simulink model "Physical_architecture"  (R2023b)
settings: Solver=VariableStepAuto  StartTime=0.0  StopTime=10.0  RelTol=1e-3
settings Model: Creator=Cristian  LastModifiedBy=Cristian

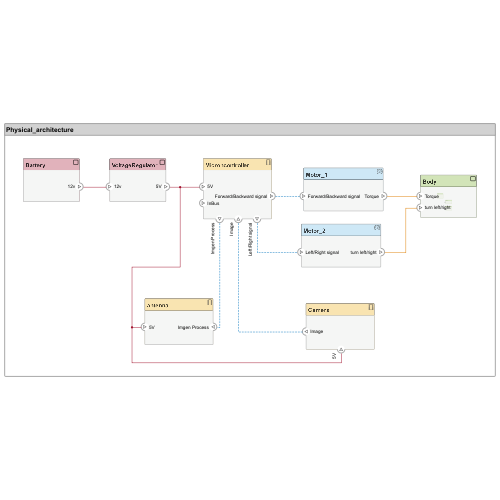
[thumbnail: Simulink's stored preview of the top-level diagram]
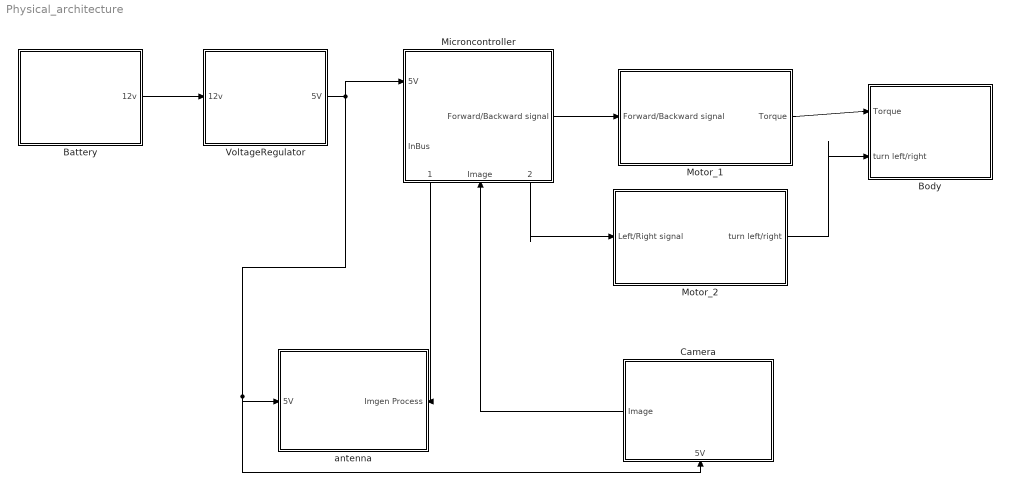
== system Physical_architecture ==
  Battery : Subsystem
      settings: PortSchema="{\"entries\":[{\"content\":{\"headerSize\":26,\"margin\":15,\"minimumSpacing\":25,\"sides\":[{\"content\":{},\"type\":\"ConnectorPlacement.EquallySpacedRectSide\",\"uuid\":\"a4c63610-ce53-4263-bc32-11f7e141828d\"},{\"content\":{\"connectorIds\":[\"Out1\"],\"side\":\"RIGHT\"},\"type\":\"ConnectorPlacement.EquallySpacedRectSide\",\"uuid\":\"7388023e-6661-4314-a5ba-fe6a68600945\"},{\"content\":{\"side\":\"TOP\"},\"type\":\"ConnectorPlacement.EquallySpacedRectSide\",\"uuid\":\"a8a6465a-b279-4272-9cd6-de33cf491c4f\"}]},\"type\":\"ConnectorPlacement.EquallySpacedConnector\",\"uuid\":\"83902977-a181-41b3-bc45-d69d98624d59\"}],\"packageUris\":[\"http://schema.mathworks.com/mf0/Connector/R2020b\"],\"version\":\"1.0\"}"
  Body : Subsystem
      settings: PortSchema="{\"entries\":[{\"content\":{\"headerSize\":26,\"margin\":15,\"minimumSpacing\":25,\"sides\":[{\"content\":{\"connectorIds\":[\"In2\",\"In1\"]},\"type\":\"ConnectorPlacement.EquallySpacedRectSide\",\"uuid\":\"a4c63610-ce53-4263-bc32-11f7e141828d\"},{\"content\":{\"side\":\"RIGHT\"},\"type\":\"ConnectorPlacement.EquallySpacedRectSide\",\"uuid\":\"7388023e-6661-4314-a5ba-fe6a68600945\"},{\"content\":{\"side\":\"TOP\"},\"type\":\"ConnectorPlacement.EquallySpacedRectSide\",\"uuid\":\"a8a6465a-b279-4272-9cd6-de33cf491c4f\"},{\"content\":{\"side\":\"BOTTOM\"},\"type\":\"ConnectorPlacement.EquallySpacedRectSide\",\"uuid\":\"22874e39-900b-4eaf-ad8f-1ca0f898979d\"}]},\"type\":\"ConnectorPlacement.EquallySpacedConnector\",\"uuid\":\"83902977-a181-41b3-bc45-d69d98624d59\"}],\"packageUris\":[\"http://schema.mathworks.com/mf0/Connector/R2020b\"],\"version\":\"1.0\"}"
  Camera : Subsystem
      settings: PortSchema="{\"entries\":[{\"content\":{\"headerSize\":26,\"margin\":15,\"minimumSpacing\":25,\"sides\":[{\"content\":{\"connectorIds\":[\"Out1\"]},\"type\":\"ConnectorPlacement.EquallySpacedRectSide\",\"uuid\":\"a4c63610-ce53-4263-bc32-11f7e141828d\"},{\"content\":{\"side\":\"RIGHT\"},\"type\":\"ConnectorPlacement.EquallySpacedRectSide\",\"uuid\":\"7388023e-6661-4314-a5ba-fe6a68600945\"},{\"content\":{\"side\":\"TOP\"},\"type\":\"ConnectorPlacement.EquallySpacedRectSide\",\"uuid\":\"a8a6465a-b279-4272-9cd6-de33cf491c4f\"},{\"content\":{\"connectorIds\":[\"In1\"],\"side\":\"BOTTOM\"},\"type\":\"ConnectorPlacement.EquallySpacedRectSide\",\"uuid\":\"23249c11-1fad-4353-8010-062f6ccc5b3b\"}]},\"type\":\"ConnectorPlacement.EquallySpacedConnector\",\"uuid\":\"83902977-a181-41b3-bc45-d69d98624d59\"}],\"packageUris\":[\"http://schema.mathworks.com/mf0/Connector/R2020b\"],\"version\":\"1.0\"}"
  Microncontroller : Subsystem
      settings: PortSchema="{\"entries\":[{\"content\":{\"headerSize\":26,\"margin\":15,\"minimumSpacing\":25,\"sides\":[{\"content\":{\"connectorIds\":[\"In2\",\"In3\"]},\"type\":\"ConnectorPlacement.EquallySpacedRectSide\",\"uuid\":\"a4c63610-ce53-4263-bc32-11f7e141828d\"},{\"content\":{\"connectorIds\":[\"Out3\"],\"side\":\"RIGHT\"},\"type\":\"ConnectorPlacement.EquallySpacedRectSide\",\"uuid\":\"7388023e-6661-4314-a5ba-fe6a68600945\"},{\"content\":{\"side\":\"TOP\"},\"type\":\"ConnectorPlacement.EquallySpacedRectSide\",\"uuid\":\"a8a6465a-b279-4272-9cd6-de33cf491c4f\"},{\"content\":{\"connectorIds\":[\"Out1\",\"In1\",\"Out2\"],\"side\":\"BOTTOM\"},\"type\":\"ConnectorPlacement.EquallySpacedRectSide\",\"uuid\":\"9aefb96e-8b5c-4ea9-bd4f-4224df175b07\"}]},\"type\":\"ConnectorPlacement.EquallySpacedConnector\",\"uuid\":\"83902977-a181-41b3-bc45-d69d98624d59\"}],\"packageUris\":[\"http://schema.mathworks.com/mf0/Connector/R2020b\"],\"version\":\"1.0\"}"
  Motor_1 : Subsystem
      settings: PortSchema="{\"entries\":[{\"content\":{\"headerSize\":26,\"margin\":15,\"minimumSpacing\":25,\"sides\":[{\"content\":{\"connectorIds\":[\"In1\"]},\"type\":\"ConnectorPlacement.EquallySpacedRectSide\",\"uuid\":\"a4c63610-ce53-4263-bc32-11f7e141828d\"},{\"content\":{\"connectorIds\":[\"Out1\"],\"side\":\"RIGHT\"},\"type\":\"ConnectorPlacement.EquallySpacedRectSide\",\"uuid\":\"7388023e-6661-4314-a5ba-fe6a68600945\"},{\"content\":{\"side\":\"TOP\"},\"type\":\"ConnectorPlacement.EquallySpacedRectSide\",\"uuid\":\"a8a6465a-b279-4272-9cd6-de33cf491c4f\"}]},\"type\":\"ConnectorPlacement.EquallySpacedConnector\",\"uuid\":\"83902977-a181-41b3-bc45-d69d98624d59\"}],\"packageUris\":[\"http://schema.mathworks.com/mf0/Connector/R2020b\"],\"version\":\"1.0\"}"
  Motor_2 : Subsystem
      settings: PortSchema="{\"entries\":[{\"content\":{\"headerSize\":26,\"margin\":15,\"minimumSpacing\":25,\"sides\":[{\"content\":{\"connectorIds\":[\"In1\"]},\"type\":\"ConnectorPlacement.EquallySpacedRectSide\",\"uuid\":\"a4c63610-ce53-4263-bc32-11f7e141828d\"},{\"content\":{\"connectorIds\":[\"Out1\"],\"side\":\"RIGHT\"},\"type\":\"ConnectorPlacement.EquallySpacedRectSide\",\"uuid\":\"7388023e-6661-4314-a5ba-fe6a68600945\"},{\"content\":{\"side\":\"TOP\"},\"type\":\"ConnectorPlacement.EquallySpacedRectSide\",\"uuid\":\"a8a6465a-b279-4272-9cd6-de33cf491c4f\"}]},\"type\":\"ConnectorPlacement.EquallySpacedConnector\",\"uuid\":\"83902977-a181-41b3-bc45-d69d98624d59\"}],\"packageUris\":[\"http://schema.mathworks.com/mf0/Connector/R2020b\"],\"version\":\"1.0\"}"
  VoltageRegulator : Subsystem
      settings: PortSchema="{\"entries\":[{\"content\":{\"headerSize\":26,\"margin\":15,\"minimumSpacing\":25,\"sides\":[{\"content\":{\"connectorIds\":[\"In1\"]},\"type\":\"ConnectorPlacement.EquallySpacedRectSide\",\"uuid\":\"a4c63610-ce53-4263-bc32-11f7e141828d\"},{\"content\":{\"connectorIds\":[\"Out1\"],\"side\":\"RIGHT\"},\"type\":\"ConnectorPlacement.EquallySpacedRectSide\",\"uuid\":\"7388023e-6661-4314-a5ba-fe6a68600945\"},{\"content\":{\"side\":\"TOP\"},\"type\":\"ConnectorPlacement.EquallySpacedRectSide\",\"uuid\":\"a8a6465a-b279-4272-9cd6-de33cf491c4f\"}]},\"type\":\"ConnectorPlacement.EquallySpacedConnector\",\"uuid\":\"83902977-a181-41b3-bc45-d69d98624d59\"}],\"packageUris\":[\"http://schema.mathworks.com/mf0/Connector/R2020b\"],\"version\":\"1.0\"}"
  antenna : Subsystem
      settings: PortSchema="{\"entries\":[{\"content\":{\"headerSize\":26,\"margin\":15,\"minimumSpacing\":25,\"sides\":[{\"content\":{\"connectorIds\":[\"In2\"]},\"type\":\"ConnectorPlacement.EquallySpacedRectSide\",\"uuid\":\"a4c63610-ce53-4263-bc32-11f7e141828d\"},{\"content\":{\"connectorIds\":[\"In1\"],\"side\":\"RIGHT\"},\"type\":\"ConnectorPlacement.EquallySpacedRectSide\",\"uuid\":\"7388023e-6661-4314-a5ba-fe6a68600945\"},{\"content\":{\"side\":\"TOP\"},\"type\":\"ConnectorPlacement.EquallySpacedRectSide\",\"uuid\":\"a8a6465a-b279-4272-9cd6-de33cf491c4f\"}]},\"type\":\"ConnectorPlacement.EquallySpacedConnector\",\"uuid\":\"83902977-a181-41b3-bc45-d69d98624d59\"}],\"packageUris\":[\"http://schema.mathworks.com/mf0/Connector/R2020b\"],\"version\":\"1.0\"}"
  wires:
  Battery/1(12v) -> VoltageRegulator/1(12v)
  VoltageRegulator/1(5V) -> antenna/2(5V), Camera/1(5V), Microncontroller/2(5V)
  Microncontroller/3(Forward/Backward signal) -> Motor_1/1(Forward/Backward signal)
  Microncontroller/2(Left/Right signal) -> Motor_2/1(Left/Right signal)
  Motor_1/1(Torque) -> Body/2(Torque)
  Motor_2/1(turn left/right) -> Body/1(turn left/right)
  Camera/1(Image) -> Microncontroller/1(Image)
  Microncontroller/1(Imgen Process) -> antenna/1(Imgen Process)

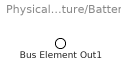
== system Physical_architecture/Battery ==
  Bus Element Out1 : Outport  PortName=12v

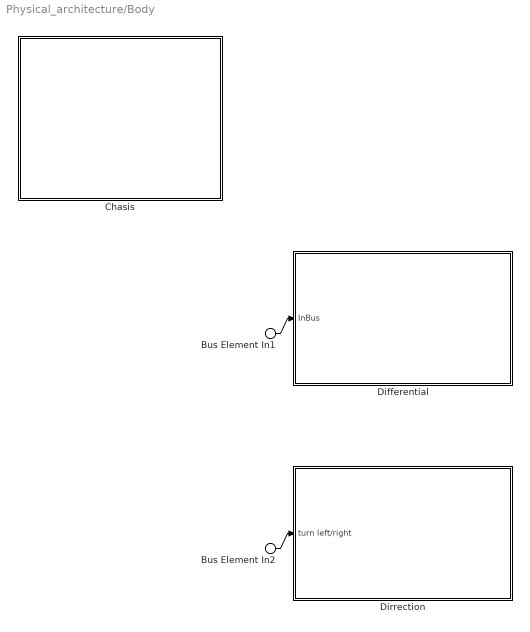
== system Physical_architecture/Body ==
  Bus Element In2 : Inport  PortName=turn left/right
  Bus Element In1 : Inport  Port=2  PortName=Torque
  Chasis : Subsystem
      settings: PortSchema="{\"entries\":[{\"content\":{\"headerSize\":26,\"margin\":15,\"minimumSpacing\":25,\"sides\":[{\"content\":{},\"type\":\"ConnectorPlacement.EquallySpacedRectSide\",\"uuid\":\"a4c63610-ce53-4263-bc32-11f7e141828d\"},{\"content\":{\"side\":\"RIGHT\"},\"type\":\"ConnectorPlacement.EquallySpacedRectSide\",\"uuid\":\"7388023e-6661-4314-a5ba-fe6a68600945\"},{\"content\":{\"side\":\"TOP\"},\"type\":\"ConnectorPlacement.EquallySpacedRectSide\",\"uuid\":\"a8a6465a-b279-4272-9cd6-de33cf491c4f\"}]},\"type\":\"ConnectorPlacement.EquallySpacedConnector\",\"uuid\":\"83902977-a181-41b3-bc45-d69d98624d59\"}],\"packageUris\":[\"http://schema.mathworks.com/mf0/Connector/R2020b\"],\"version\":\"1.0\"}"
  Differential : Subsystem
      settings: PortSchema="{\"entries\":[{\"content\":{\"headerSize\":26,\"margin\":15,\"minimumSpacing\":25,\"sides\":[{\"content\":{\"connectorIds\":[\"In1\"]},\"type\":\"ConnectorPlacement.EquallySpacedRectSide\",\"uuid\":\"a4c63610-ce53-4263-bc32-11f7e141828d\"},{\"content\":{\"side\":\"RIGHT\"},\"type\":\"ConnectorPlacement.EquallySpacedRectSide\",\"uuid\":\"7388023e-6661-4314-a5ba-fe6a68600945\"},{\"content\":{\"side\":\"TOP\"},\"type\":\"ConnectorPlacement.EquallySpacedRectSide\",\"uuid\":\"a8a6465a-b279-4272-9cd6-de33cf491c4f\"}]},\"type\":\"ConnectorPlacement.EquallySpacedConnector\",\"uuid\":\"83902977-a181-41b3-bc45-d69d98624d59\"}],\"packageUris\":[\"http://schema.mathworks.com/mf0/Connector/R2020b\"],\"version\":\"1.0\"}"
  Dirrection : Subsystem
      settings: PortSchema="{\"entries\":[{\"content\":{\"headerSize\":26,\"margin\":15,\"minimumSpacing\":25,\"sides\":[{\"content\":{\"connectorIds\":[\"In1\"]},\"type\":\"ConnectorPlacement.EquallySpacedRectSide\",\"uuid\":\"a4c63610-ce53-4263-bc32-11f7e141828d\"},{\"content\":{\"side\":\"RIGHT\"},\"type\":\"ConnectorPlacement.EquallySpacedRectSide\",\"uuid\":\"7388023e-6661-4314-a5ba-fe6a68600945\"},{\"content\":{\"side\":\"TOP\"},\"type\":\"ConnectorPlacement.EquallySpacedRectSide\",\"uuid\":\"a8a6465a-b279-4272-9cd6-de33cf491c4f\"}]},\"type\":\"ConnectorPlacement.EquallySpacedConnector\",\"uuid\":\"83902977-a181-41b3-bc45-d69d98624d59\"}],\"packageUris\":[\"http://schema.mathworks.com/mf0/Connector/R2020b\"],\"version\":\"1.0\"}"
  wires:
  Bus Element In1/1 -> Differential/1(InBus)
  Bus Element In2/1 -> Dirrection/1(turn left/right)

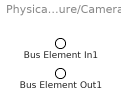
== system Physical_architecture/Camera ==
  Bus Element In1 : Inport  PortName=5V
  Bus Element Out1 : Outport  PortName=Image

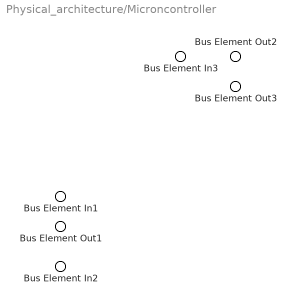
== system Physical_architecture/Microncontroller ==
  Bus Element In3 : Inport  PortName=Image
  Bus Element In1 : Inport  Port=2  PortName=5V
  Bus Element In2 : Inport  Port=3  PortName=InBus
  Bus Element Out3 : Outport  PortName=Imgen Process
  Bus Element Out2 : Outport  Port=2  PortName=Left/Right signal
  Bus Element Out1 : Outport  Port=3  PortName=Forward/Backward signal

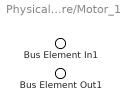
== system Physical_architecture/Motor_1 ==
  Bus Element In1 : Inport  PortName=Forward/Backward signal
  Bus Element Out1 : Outport  PortName=Torque

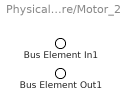
== system Physical_architecture/Motor_2 ==
  Bus Element In1 : Inport  PortName=Left/Right signal
  Bus Element Out1 : Outport  PortName=turn left/right

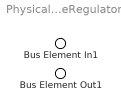
== system Physical_architecture/VoltageRegulator ==
  Bus Element In1 : Inport  PortName=12v
  Bus Element Out1 : Outport  PortName=5V

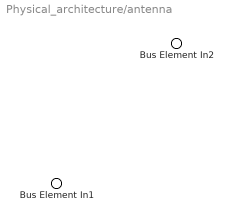
== system Physical_architecture/antenna ==
  Bus Element In2 : Inport  PortName=Imgen Process
  Bus Element In1 : Inport  Port=2  PortName=5V

== system Physical_architecture/Body/Chasis ==

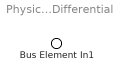
== system Physical_architecture/Body/Differential ==
  Bus Element In1 : Inport  PortName=InBus

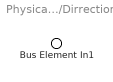
== system Physical_architecture/Body/Dirrection ==
  Bus Element In1 : Inport  PortName=turn left/right
